simulink model "vehicle_motion_model_final_temp"  (R2021b)
settings: Solver=ode5  StartTime=0.0  StopTime=600  FixedStep=0.001  RelTol=1e-3
StopFcn:
  | % stop simulation callback function
  | figure(1);
  | out.x_gt.data = permute(out.x_gt.data,[3, 1, 2]);
  | plot3(out.x_gt.data(:, 1), out.x_gt.data(:, 2), -out.x_gt.data(:, 3), 'Color', 'r', 'LineWidth', 1.5);
  | legend('Истинная траектория')
  | xlabel('X, \itм');
  | ylabel('Y, \itм');
  | zlabel('Z, \itм');
  | figure(2);
  | plot3(out.x.data(:, 1), out.x.data(:, 2), -out.x.data(:, 3), 'Color', 'b', 'LineWidth', 1.5);
  | hold on;
  | xlabel('X, \itм');
  | ylabel('Y, \itм');
  | zlabel('Z, \itм');
  | % legend('pos')
  | hold on;
  | plot3(out.x_gt.data(:, 1), out.x_gt.data(:, 2), -out.x_gt.data(:, 3), 'Color', 'r', 'LineWidth', 1.5);
  | hold on;
  | legend('Рассчитанная траектория', 'Истинная траектория')
  | % errors
  | figure(3);
  | yyaxis left;
  | plot(out.hor_err_fus.time, out.hor_err_fus.data, 'Color', 'b', 'LineWidth', 1.5);
  | xlabel('время, \itс');
  | ylabel('Горизонтальная ошибка, \itм');
  | hold on;
  | yyaxis right;
  | plot(out.ver_err_fus.time, out.ver_err_fus.data, 'Color', 'r', 'LineWidth', 1.5);
  | ylabel('Вертикальная ошибка, \itм');
  | legend('Горизонтальная позиционная ошибка', 'Вертикальная позиционная ошибка');
  | grid on;
  | figure(4);
  | yyaxis left;
  | plot(out.hor_err_ins.time, out.hor_err_ins.data, '-', 'Color', 'b', 'LineWidth', 1.5);
  | xlabel('время, \itс');
  | ylabel('Горизонтальная ошибка, \itм');
  | hold on;
  | yyaxis right;
  | plot(out.ver_err_ins.time, out.ver_err_ins.data, '-', 'Color', 'r', 'LineWidth', 1.5);
  | ylabel('Вертикальная ошибка, \itм');
  | legend('Горизонтальная позиционная ошибка', 'Вертикальная позиционная ошибка');
  | grid on;
model workspace (MAT data in the model file):
  AxlIxx = 62.3745166667
  AxlM = 160
  Cps = 2
  CzWhlAxl = 557955.087061
  DCT_Param : object (value not decoded)
  Downshift_Speeds = [9.5625 12.9375 16.3125 19.6875 23.0625 26.4375 29.8125 33.1875 36.5625 39.9375 43.3125 46.6875 ... (28 elements, 4x7)]
  F0zWhlAxl = 16132.2380068
  HTCH : object (value not decoded)
  Hmax = 0.25
  KzWhlAxl = 58428920.0848
  NCyl = 6
  Pedal_Positions = [0.1 0.4 0.5 0.9]
  Pstd = 101325
  Q = [1  0  0; 0  1  0; 0  0  1]
  Rair = 287
  SUS : object (value not decoded)
  TRA : object (value not decoded)
  Trans : object (value not decoded)
  Tstd = 293.15
  Upshift_Speeds = [12.9375 16.3125 19.6875 33 26.4375 29.8125 33.1875 52.5 39.9375 43.3125 46.6875 77.25 ... (28 elements, 4x7)]
  VEH : object (value not decoded)
  Vd = 0.00346
  WH : Mass (value not decoded)
  dt3D = 0.05
  f_air = [0 0 0 0 0 0 0 0 0 0 0 0 ... (256 elements, 16x16)]
  f_co = [0 0 0 0 0 0 0 0 0 0 0 0 ... (256 elements, 16x16)]
  f_co2 = [0 0 0 0 0 0 0 0 0 0 0 0 ... (256 elements, 16x16)]
  f_eff = [352.135682859 352.135682859 320.724378192 303.655312657 295.930136708 291.240087194 291.240271258 291.240312459 291.240275452 291.240198499 291.240100781 291.240018769 ... (256 elements, 16x16)]
  f_fuel = [0 0 0 0 0 0 0 0 0 0 0 0 ... (256 elements, 16x16)]
  f_hc = [0 0 0 0 0 0 0 0 0 0 0 0 ... (256 elements, 16x16)]
  f_nox = [0 0 0 0 0 0 0 0 0 0 0 0 ... (256 elements, 16x16)]
  f_pm = [0 0 0 0 0 0 0 0 0 0 0 0 ... (256 elements, 16x16)]
  f_susp_axl_bp = [1 2]
  f_susp_dz_bp = [-0.325022776267 -0.315022776267 -0.305022776267 -0.205022776267 -0.105022776267 -0.00502277626717 0.0949772237328 0.194977223733 0.204977223733 0.214977223733]
  f_susp_dzdot_bp = [-3 -0.3 -0.2 -0.1 0 0.1 0.2 0.3 3]
  f_susp_fmz = [-144070.391448 -93629.24037 -75929.1118915 -20630.5828179 -15385.48216 -10140.3815021 -4895.28084414 349.819813785 -31916.3973792 18437.6709544 -83996.1993354 -33555.0482577 ... (43920 elements, 10x9x61x2x4)]
  f_susp_geom = [0 0 0 0 0 0 0 0 0 0 0 0 ... (3660 elements, 10x61x2x3)]
  f_susp_strgdelta_bp = [-0.523598775598 -0.506145483078 -0.488692190558 -0.471238898038 -0.453785605519 -0.436332312999 -0.418879020479 -0.401425727959 -0.383972435439 -0.366519142919 -0.349065850399 -0.331612557879 ... (61 elements, 1x61)]
  f_tbrake = [0 76.8593923996 105.140482948 131.533638111 157.926793274 176.658631717 176.65727296 176.656856686 176.656879077 176.657093756 176.657404516 176.65772406 ... (256 elements, 16x16)]
  f_tbrake_n_bpt = [0 649.519052838 912.419621844 1175.32019085 1438.22075986 1701.12132886 1964.02189787 2226.92246687 2489.82303588 2752.72360489 3015.62417389 3278.5247429 ... (16 elements, 1x16)]
  f_tbrake_t_bpt = [0 34.6410161514 61.0341713143 87.4273264773 113.82048164 140.213636803 166.606791966 192.999947129 219.393102292 245.786257455 272.179412618 298.572567781 ... (16 elements, 1x16)]
  f_texh = [766.752464599 766.752464599 786.17542386 801.679939032 884.591982581 910.574397722 910.571871054 910.570774534 910.570601632 910.570821151 910.571247242 910.571639815 ... (256 elements, 16x16)]
  f_twc_eff_co = [0.17 0.25 0.45 0.99 0.99 0.99 0.99]
  f_twc_eff_hc = [0.21 0.375 0.75 0.98 0.98 0.98 0.98]
  f_twc_eff_lam = [0.909090909 0.944055944 0.979020979 1 1.013986014 1.048951049 1.083916084]
  f_twc_eff_nox = [0.98 0.98 0.98 0.97 0.05 0.02 0]
  h = 0.134
symbols that are objects in the model workspace (value not decoded): VEH
libraries: aerolibcommonsys x8, sharedtransform x8, sharedutil x7, autolibsharedcommon x7, autolibutils x4, vehdynlibtirecommon x3, dspstat3 x2, mspsensorlib x1, aerolibnav x1, shared6dof x1, autolibshared x1, vehdynlibsuspension x1
(part 9 of 9)

== matlab function vehicle_motion_model_final_temp/Two-Axle Vehicle/Wheels and Tires/Wheels and Tires/Tires/MF Tires/Combined Slip Wheel 2DOF/Magic Tire Const Input/Magic Tire Const Input ==
  data: Omega input; Vx input; Vy input; psidot input; Gamma input; TirePrs input; ScaleFactors input; rhoz input; plySteer parameter; Fx output; Fy output double; FzTire output; Mx output; My output; Mz output; Re output; Kappa output; Alpha output; sig_x output; sig_y output; PRESMAX parameter; PRESMIN parameter; FZMAX parameter; FZMIN parameter; VXLOW parameter; KPUMAX parameter; KPUMIN parameter; ALPMAX parameter; ALPMIN parameter; CAMMIN parameter; CAMMAX parameter; LONGVL parameter; UNLOADED_RADIUS parameter; RIM_RADIUS parameter; NOMPRES parameter; FNOMIN parameter; VERTICAL_STIFFNESS parameter; DREFF parameter; BREFF parameter; FREFF parameter; Q_RE0 parameter; Q_V1 parameter; Q_V2 parameter; Q_FZ1 parameter; Q_FZ2 parameter; Q_FCX parameter; Q_FCY parameter; PFZ1 parameter; Q_FCY2 parameter; BOTTOM_OFFST parameter; BOTTOM_STIFF parameter; PCX1 parameter; PDX1 parameter; PDX2 parameter; PDX3 parameter; PEX1 parameter; PEX2 parameter; PEX3 parameter; PEX4 parameter; PKX1 parameter; PKX2 parameter; PKX3 parameter; PHX1 parameter; PHX2 parameter; PVX1 parameter; PVX2 parameter; PPX1 parameter; PPX2 parameter; PPX3 parameter; PPX4 parameter; RBX1 parameter; RBX2 parameter; RBX3 parameter; RCX1 parameter; REX1 parameter; REX2 parameter; RHX1 parameter; QSX1 parameter; QSX2 parameter; QSX3 parameter; QSX4 parameter; QSX5 parameter; QSX6 parameter; QSX7 parameter; QSX8 parameter; QSX9 parameter; QSX10 parameter; QSX11 parameter; PPMX1 parameter; PCY1 parameter; PDY1 parameter; PDY2 parameter; PDY3 parameter; PEY1 parameter; PEY2 parameter; PEY3 parameter; PEY4 parameter; PEY5 parameter; PKY1 parameter; PKY2 parameter; PKY3 parameter; PKY4 parameter; PKY5 parameter; PKY6 parameter; PKY7 parameter; PHY1 parameter; PHY2 parameter; PVY1 parameter; PVY2 parameter; PVY3 parameter; PVY4 parameter; PPY1 parameter; PPY2 parameter; PPY3 parameter; PPY4 parameter; PPY5 parameter; RBY1 parameter; RBY2 parameter; RBY3 parameter; RBY4 parameter; RCY1 parameter; REY1 parameter; REY2 parameter; RHY1 parameter; RHY2 parameter; RVY1 parameter; RVY2 parameter; RVY3 parameter; RVY4 parameter; RVY5 parameter; RVY6 parameter; QSY1 parameter; QSY2 parameter; QSY3 parameter; QSY4 parameter; QSY5 parameter; QSY6 parameter; QSY7 parameter; QSY8 parameter; QBZ1 parameter; QBZ2 parameter; QBZ3 parameter; QBZ4 parameter; QBZ5 parameter; QBZ6 parameter; QBZ9 parameter; QBZ10 parameter; QCZ1 parameter; QDZ1 parameter; QDZ2 parameter; QDZ3 parameter; QDZ4 parameter; QDZ6 parameter; QDZ7 parameter; QDZ8 parameter; QDZ9 parameter; QDZ10 parameter; QDZ11 parameter; QEZ1 parameter; QEZ2 parameter; QEZ3 parameter; QEZ4 parameter; QEZ5 parameter; QHZ1 parameter; QHZ2 parameter; QHZ3 parameter; QHZ4 parameter; PPZ1 parameter; PPZ2 parameter; SSZ1 parameter; SSZ2 parameter; SSZ3 parameter; SSZ4 parameter; PDXP1 parameter; PDXP2 parameter; PDXP3 parameter; PKYP1 parameter; PDYP1 parameter; PDYP2 parameter; PDYP3 parameter; PDYP4 parameter; PHYP1 parameter; PHYP2 parameter; PHYP3 parameter; PHYP4 parameter; PECP1 parameter; PECP2 parameter; QDTP1 parameter; QCRP1 parameter; QCRP2 parameter; QBRP1 parameter; QDRP1 parameter; QDRP2 parameter; WIDTH parameter; Q_RA1 parameter; Q_RA2 parameter; Q_RB1 parameter; Q_RB2 parameter; QSX12 parameter; QSX13 parameter; QSX14 parameter; a output; b output; Q_FZ3 parameter; LONGITUDINAL_STIFFNESS parameter; LATERAL_STIFFNESS parameter; PCFX1 parameter; PCFX2 parameter; PCFX3 parameter; PCFY1 parameter; PCFY2 parameter; PCFY3 parameter; Fx_ext input; Fy_ext input; vdynMF parameter size=279
% Copyright 2018-2021 The MathWorks, Inc.
function [Fx,Fy,FzTire,Mx,My,Mz,Re,Kappa,Alpha,sig_x,sig_y,a,b] = magictire(Omega,Vx,Vy,psidot,Gamma,TirePrs,ScaleFactors,rhoz,plySteer,...
    PRESMAX,...
    PRESMIN,...
    FZMAX,...
    FZMIN,...
    VXLOW,...
    KPUMAX,...
    KPUMIN,...
    ALPMAX,...
    ALPMIN,...
    CAMMIN,...
    CAMMAX,...
    LONGVL,...
    UNLOADED_RADIUS,...    
    RIM_RADIUS,...
    NOMPRES,...
    FNOMIN,...
    VERTICAL_STIFFNESS,...% vertical
    DREFF,...
    BREFF,...
    FREFF,...
    Q_RE0,...
    Q_V1,...
    Q_V2,...
    Q_FZ1,...
    Q_FZ2,...
    Q_FCX,...
    Q_FCY,...
    PFZ1,...
    Q_FCY2,...
    BOTTOM_OFFST,...
    BOTTOM_STIFF,...
    PCX1,...% longitudinal
    PDX1,...
    PDX2,...
    PDX3,...
    PEX1,...
    PEX2,...
    PEX3,...
    PEX4,...
    PKX1,...
    PKX2,...
    PKX3,...
    PHX1,...
    PHX2,...
    PVX1,...
    PVX2,...
    PPX1,...
    PPX2,...
    PPX3,...
    PPX4,...
    RBX1,...
    RBX2,...
    RBX3,...
    RCX1,...
    REX1,...
    REX2,...
    RHX1,...
    QSX1,...% overturning
    QSX2,...
    QSX3,...
    QSX4,...
    QSX5,...
    QSX6,...
    QSX7,...
    QSX8,...
    QSX9,...
    QSX10,...
    QSX11,...
    PPMX1,...
    PCY1,...% lateral
    PDY1,...
    PDY2,...
    PDY3,...
    PEY1,...
    PEY2,...
    PEY3,...
    PEY4,...
    PEY5,...
    PKY1,...
    PKY2,...
    PKY3,...
    PKY4,...
    PKY5,...
    PKY6,...
    PKY7,...
    PHY1,...
    PHY2,...
    PVY1,...
    PVY2,...
    PVY3,...
    PVY4,...
    PPY1,...
    PPY2,...
    PPY3,...
    PPY4,...
    PPY5,...
    RBY1,...
    RBY2,...
    RBY3,...
    RBY4,...
    RCY1,...
    REY1,...
    REY2,...
    RHY1,...
    RHY2,...
    RVY1,...
    RVY2,...
    RVY3,...
    RVY4,...
    RVY5,...
    RVY6,...
    QSY1,...% rolling
    QSY2,...
    QSY3,...
    QSY4,...
    QSY5,...
    QSY6,...
    QSY7,...
    QSY8,...
    QBZ1,...
    QBZ2,...
    QBZ3,...
    QBZ4,...
    QBZ5,...
    QBZ6,...
    QBZ9,...
    QBZ10,...
    QCZ1,...
    QDZ1,...
    QDZ2,...
    QDZ3,...
    QDZ4,...
    QDZ6,...
    QDZ7,...
    QDZ8,...
    QDZ9,...
    QDZ10,...
    QDZ11,...
    QEZ1,...
    QEZ2,...
    QEZ3,...
    QEZ4,...
    QEZ5,...
    QHZ1,...
    QHZ2,...
    QHZ3,...
    QHZ4,...
    PPZ1,...
    PPZ2,...
    SSZ1,...
    SSZ2,...
    SSZ3,...
    SSZ4,...
    PDXP1,...% turn slip
    PDXP2,...
    PDXP3,...
    PKYP1,...
    PDYP1,...
    PDYP2,...
    PDYP3,...
    PDYP4,...
    PHYP1,...
    PHYP2,...
    PHYP3,...
    PHYP4,...
    PECP1,...
    PECP2,...
    QDTP1,...
    QCRP1,...% aligning moment
    QCRP2,...
    QBRP1,...
    QDRP1,...
    QDRP2,...
    WIDTH,...
    Q_RA1,... % contact patch
    Q_RA2,...
    Q_RB1,...
    Q_RB2,...
    QSX12,...
    QSX13,...
    QSX14,...
    Q_FZ3,...
    LONGITUDINAL_STIFFNESS,...% structural
    LATERAL_STIFFNESS,...
    PCFX1,...
    PCFX2,...
    PCFX3,...
    PCFY1,...
    PCFY2,...
    PCFY3,...
    Fx_ext,...
    Fy_ext,...
    vdynMF)...
%#codegen
coder.allowpcode('plain')
[Fx,Fy,FzTire,Mx,My,Mz,Re,Kappa,Alpha,sig_x,sig_y,a,b] = vdyncsmtire(Omega,Vx,Vy,psidot,Gamma,TirePrs,ScaleFactors,rhoz,plySteer,...
    PRESMAX,...
    PRESMIN,...
    FZMAX,...
    FZMIN,...
    VXLOW,...
    KPUMAX,...
    KPUMIN,...
    ALPMAX,...
    ALPMIN,...
    CAMMIN,...
    CAMMAX,...
    LONGVL,...
    UNLOADED_RADIUS,...
    RIM_RADIUS,...
    NOMPRES,...
    FNOMIN,...
    VERTICAL_STIFFNESS,...% vertical
    DREFF,...
    BREFF,...
    FREFF,...
    Q_RE0,...
    Q_V1,...
    Q_V2,...
    Q_FZ1,...
    Q_FZ2,...
    Q_FCX,...
    Q_FCY,...
    PFZ1,...
    Q_FCY2,...
    BOTTOM_OFFST,...
    BOTTOM_STIFF,...
    PCX1,...% longitudinal
    PDX1,...
    PDX2,...
    PDX3,...
    PEX1,...
    PEX2,...
    PEX3,...
    PEX4,...
    PKX1,...
    PKX2,...
    PKX3,...
    PHX1,...
    PHX2,...
    PVX1,...
    PVX2,...
    PPX1,...
    PPX2,...
    PPX3,...
    PPX4,...
    RBX1,...
    RBX2,...
    RBX3,...
    RCX1,...
    REX1,...
    REX2,...
    RHX1,...
    QSX1,...% overturning
    QSX2,...
    QSX3,...
    QSX4,...
    QSX5,...
    QSX6,...
    QSX7,...
    QSX8,...
    QSX9,...
    QSX10,...
    QSX11,...
    PPMX1,...
    PCY1,...% lateral
    PDY1,...
    PDY2,...
    PDY3,...
    PEY1,...
    PEY2,...
    PEY3,...
    PEY4,...
    PEY5,...
    PKY1,...
    PKY2,...
    PKY3,...
    PKY4,...
    PKY5,...
    PKY6,...
    PKY7,...
    PHY1,...
    PHY2,...
    PVY1,...
    PVY2,...
    PVY3,...
    PVY4,...
    PPY1,...
    PPY2,...
    PPY3,...
    PPY4,...
    PPY5,...
    RBY1,...
    RBY2,...
    RBY3,...
    RBY4,...
    RCY1,...
    REY1,...
    REY2,...
    RHY1,...
    RHY2,...
    RVY1,...
    RVY2,...
    RVY3,...
    RVY4,...
    RVY5,...
    RVY6,...
    QSY1,...% rolling
    QSY2,...
    QSY3,...
    QSY4,...
    QSY5,...
    QSY6,...
    QSY7,...
    QSY8,...
    QBZ1,...
    QBZ2,...
    QBZ3,...
    QBZ4,...
    QBZ5,...
    QBZ6,...
    QBZ9,...
    QBZ10,...
    QCZ1,...
    QDZ1,...
    QDZ2,...
    QDZ3,...
    QDZ4,...
    QDZ6,...
    QDZ7,...
    QDZ8,...
    QDZ9,...
    QDZ10,...
    QDZ11,...
    QEZ1,...
    QEZ2,...
    QEZ3,...
    QEZ4,...
    QEZ5,...
    QHZ1,...
    QHZ2,...
    QHZ3,...
    QHZ4,...
    PPZ1,...
    PPZ2,...
    SSZ1,...
    SSZ2,...
    SSZ3,...
    SSZ4,...
    PDXP1,...% turn slip
    PDXP2,...
    PDXP3,...
    PKYP1,...
    PDYP1,...
    PDYP2,...
    PDYP3,...
    PDYP4,...
    PHYP1,...
    PHYP2,...
    PHYP3,...
    PHYP4,...
    PECP1,...
    PECP2,...
    QDTP1,...
    QCRP1,...% aligning moment
    QCRP2,...
    QBRP1,...
    QDRP1,...
    QDRP2,...
    WIDTH,...
    Q_RA1,... % contact patch
    Q_RA2,...
    Q_RB1,...
    Q_RB2,...
    QSX12,...
    QSX13,...
    QSX14,...
    Q_FZ3,...
    LONGITUDINAL_STIFFNESS,...% structural
    LATERAL_STIFFNESS,...
    PCFX1,...
    PCFX2,...
    PCFX3,...
    PCFY1,...
    PCFY2,...
    PCFY3,...
    Fx_ext,...
    Fy_ext,...
    vdynMF);
end

== matlab function vehicle_motion_model_final_temp/BINS kinematics Euler/Turning equations ==
  data: ang input; dv_dt output; w input
function dv_dt = fcn(ang, w)
    dv_dt = Euler_motion_equation(ang, w);
end

== matlab function vehicle_motion_model_final_temp/BINS kinematics quaternion/Turning equations ==
  data: quat input; dl_dt output; w input
function dl_dt = fcn(quat, w)
    dl_dt = quatenion_motion_equation(quat, w);
end

== matlab function vehicle_motion_model_final_temp/BINS kinematics quaternion/calc begin values quater ==
  data: ang input; l output
function l = fcn(ang)
    l = quaternion_from_ang(ang);
end

== matlab function vehicle_motion_model_final_temp/BINS kinematics quaternion/DCM calc ==
  data: q input; DCM_calc output
function DCM_calc = fcn(q)
    DCM_calc = DCM_calc_from_quat(q);
end

== matlab function vehicle_motion_model_final_temp/BINS kinematics quaternion/To angles ==
  data: q input; ang output
function ang = fcn(q)
    ang = quaternion_to_angles(q);
end

== matlab function vehicle_motion_model_final_temp/Sensor fusion/Correction ==
  data: x input; x output; P output; P input; T input; z input
function [x, P] = correction(x, P, T, z)
% do correction step
    sigma_odo = 0.01;
    R = eye(3)*sigma_odo;

%     if mod(T, 5) == 0
    if mod(T, 0.1) == 0
        H_jac = DH_func();
        K = P*transpose(H_jac)*inv(H_jac*P*transpose(H_jac) + R);
        delta = K*(z - H_func(x));

        % update
        x(1:3) = x(1:3) + delta(1:3);
        x(4:6) = x(4:6) + delta(4:6);
        x(7:10) = quat_mult(quaternion_from_ang(delta(7:9)), x(7:10));
        x(11:13) = x(11:13) + delta(10:12);
        x(14:16) = x(14:16) + delta(13:15);
        x(17:19) = x(17:19) + delta(16:18);

        % compute the corrected covariance
        P = (eye(18) - K*H_jac)*P;
        
        G = eye(18);
        G(7:9, 7:9) = eye(3) - skew_symmetric(0.5*delta(7:9));
        
        P = G*P*transpose(G);
    end
end

== matlab function vehicle_motion_model_final_temp/Odometer kinimatics/MATLAB Function1 ==
  data: WhlVel input; InertFrmPos input; InertFrmAng input; omega_eb input; v_eb output; T_r input; l_br input
function v_eb = fcn(WhlVel, InertFrmPos, InertFrmAng, omega_eb, T_r, l_br)
 v_eb = odometer_kinematics(WhlVel, InertFrmPos, InertFrmAng, omega_eb, T_r, l_br);
end
    
% function v_eb = odometer_kinematics(WhlVel, InertFrmPos, InertFrmAng, omega_eb, T_r, l_br)
%     v_er = 0.5*(WhlVel(3) + WhlVel(4));
%     v_eb = [v_er; 0; 0] - skew_symmetric(omega_eb)*[-l_br; 0; 0];
% end

== matlab function vehicle_motion_model_final_temp/Calc errors2/To angles ==
  data: qat input; ang output
function ang = fcn(qat)
%#codegen
    q0 = qat(1);
    q1 = qat(2);
    q2 = qat(3);
    q3 = qat(4);
    phi = atan2(2*(q2*q3 + q0*q1), (q0^2 - q1^2 - q2^2 - q3^2));
    theta = asin(-2*(q1*q3 - q0*q2));
    psi = atan2(2*(q1*q2 +q0*q3), (q0^2 + q1^2 - q2^2 - q3^2));
    ang = [phi; theta; psi];
end

== matlab function vehicle_motion_model_final_temp/Sensor fusion/Prediction ==
  data: x_ input; x output; P output; P_ input; dT input; BINS_output input
function [x, P] = prediction(x_, P_, dT, BINS_output)
% do prediction step

    sigma_IMU_a = 0.0003;
    sigma_IMU_w = 0.00008;
    sigma_IMU_ab = 0;
    sigma_IMU_wb = 0;
    Q = eye(12);
    Q(1:3, 1:3) = sigma_IMU_a * sigma_IMU_a * Q(1:3, 1:3)*dT*dT;
    Q(4:6, 4:6) = sigma_IMU_w * sigma_IMU_w * Q(4:6, 4:6)*dT*dT;
    Q(7:9, 7:9) = sigma_IMU_ab * sigma_IMU_ab * Q(7:9, 7:9)*dT;
    Q(10:12, 10:12) = sigma_IMU_wb * sigma_IMU_wb * Q(10:12, 10:12)*dT;
    L_jac = zeros(18, 12);
    L_jac(4:15, :) = eye(12);

    % Update nominal state with IMU inputs
    x = F_func(x_, dT, BINS_output);
    % Linearize Motion Model and compute Jacobians (for the error state)
    F_jac = DF_func(x_, dT, BINS_output);
    % Propagate uncertainty
    P = F_jac*P_*transpose(F_jac) + L_jac*Q*transpose(L_jac);
end
